simulink model "Lab_Loadcell"  (R2026a)
settings: Solver=FixedStepDiscrete  StartTime=0  StopTime=inf  FixedStep=0.001
undefined symbols (not defined in the file or in its folder): Blocking, Non
libraries: amg_usbconverter_n_connect_lib x2, dspstat3 x2, dspfdesign x1
settings Model: PauseTimes=10  Creator=pboon  LastModifiedBy=bocchichan

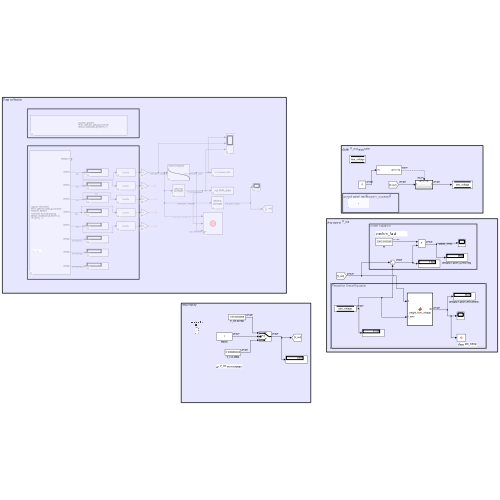
[thumbnail: Simulink's stored preview of the top-level diagram]
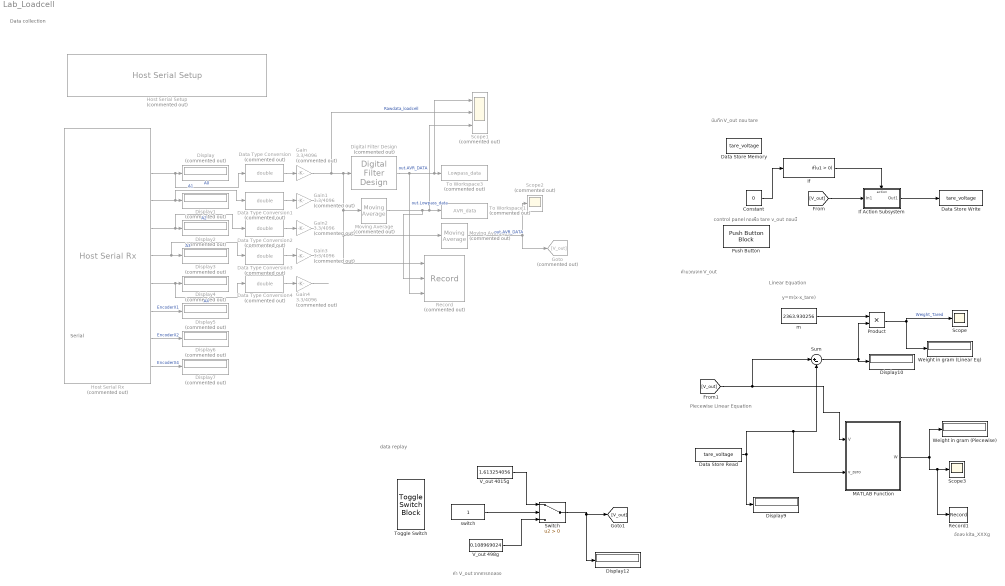
== system Lab_Loadcell ==
  note: อัดลง kita_XXXg
  note: ค่า V_out จากการทดลอง
  note: Data collection
  note: data replay
  note: Piecewise Linear Equation
  note: Linear Equation
  note: คำนวณจาก V_out
  note: control panel กดเพื่อ tare v_out ตอนนี้
  note: บันทึก V_out ตอน tare
  note: y=m(x-x_tare)
  note: Serial
  Constant : Constant  Value=0
  Data Store Memory : DataStoreMemory  DataStoreName=tare_voltage  WriteAfterWriteMsg=warning  ShowAdditionalParam=off  Dimensions=1
  Data Store Read : DataStoreRead  DataStoreName=tare_voltage  IndexOptions=Index vector (dialog)  Indices=1  OutputSizes=1
  Data Store Write : DataStoreWrite  DataStoreName=tare_voltage  IndexOptions=Index vector (dialog)  Indices=1  OutputSizes=1
  Data Type Conversion{,1..4} (5 alike) : DataTypeConversion  Commented=on  OutDataTypeStr=double  SaturateOnIntegerOverflow=off  RndMeth=Floor
  Digital Filter Design : dspfdesign/Digital Filter Design  Commented=on  mwdsp_browser_bugfix_var=off
  Display{,1..7} (8 alike) : Display  Commented=on
  Display10 : Display
  Display12 : Display
  Display9 : Display
  Gain{,1..4} (5 alike) : Gain  Commented=on  Gain=3.3/4096
  Goto : Goto  Commented=on  GotoTag=V_out
  Host Serial Rx : amg_usbconverter_n_connect_lib/Host Serial Rx  Commented=on  conf=rx  port=<auto>  baudrate=2000000  databits=8  parity=None  stopbit=1  flowcontrol=None  transfer=Non-Blocking  timeout=5  packetmode=Binary  enableinitialvalues=off  initialvalues=[]  binheader='25'  binterminator='4E 4E'  porttype_double=0  porttype_single=0  porttype_int8=0  porttype_uint8=0  porttype_int16=0  porttype_uint16=5  porttype_int32=0  porttype_uint32=3  asciiformat='%d,%f'  rx_asciiterminator="CRLF (0x0D 0x0A - \"\\r\\n\")"  tx_asciiterminator="CRLF (0x0D 0x0A - \"\\r\\n\")"  sampletime=0.001  enablecustomportlabel=off  cinputportlabel=0  coutputportlabel=A  portpinstr=0  blockid=HostSerialRx  inputporttype=[]  inputportwidth=[]  inputportlabel={}  outputporttype=[3 5 5 5 5 5 7 7 7]  outputportwidth=[1 1 1 1 1 1 1 1 1]  outputportlabel={'READY','uint16','uint16','uint16','uint16','uint16','uint32','uint32','uint32'}  compat=0  optionstring=[]  autoport='/dev/cu.debug-console'
  Host Serial Setup : amg_usbconverter_n_connect_lib/Host Serial Setup  Commented=on  conf=setup  port=<auto>  baudrate=2000000  databits=8  parity=None  stopbit=1  flowcontrol=None  transfer=Blocking  timeout=2  packetmode=Binary  initialvalues=[]  binheader='7E 7E'  binterminator='03 03'  porttype_double=0  porttype_single=1  porttype_int8=0  porttype_uint8=0  porttype_int16=0  porttype_uint16=0  porttype_int32=0  porttype_uint32=2  asciiformat='%d %u %x'  rx_asciiterminator="CRLF (0x0D 0x0A - \"\\r\\n\")"  tx_asciiterminator="CRLF (0x0D 0x0A - \"\\r\\n\")"  sampletime=-1  enablecustomportlabel=off  cinputportlabel=0  coutputportlabel=A  portpinstr=0  blockid=HostSerialSetup  inputporttype=[]  inputportwidth=[]  inputportlabel={}  outputporttype=[]  outputportwidth=[]  outputportlabel={}  compat=0  optionstring=[]  autoport='/dev/cu.debug-console'
  If : If  ShowElse=off
  If Action Subsystem : Subsystem  TreatAsAtomicUnit=on
  MATLAB Function : MATLAB Function  TreatAsAtomicUnit=on
  Moving Average : dspstat3/Moving Average  Commented=on  Method=Sliding window  ForgettingFactorPort=off  SpecifyWindowLength=on  WindowLengthSource=Property  MaxWindowLength=20  WindowLength=50  OverlapLength=49  AllowArbitraryInputLength=off  ForgettingFactor=0.9  SimulateUsing=Interpreted execution
  Moving Average1 : dspstat3/Moving Average  Commented=on  Method=Sliding window  ForgettingFactorPort=off  SpecifyWindowLength=on  WindowLengthSource=Property  MaxWindowLength=20  WindowLength=500  OverlapLength=499  AllowArbitraryInputLength=off  ForgettingFactor=0.9  SimulateUsing=Interpreted execution
  Product : Product
  Push Button : PushButtonBlock  ButtonText=Tare  IconOnColor=[0.0, 0.39215686274509803, 0.0]  IconOffColor=[0.0, 1.0, 0.0]  OffValue=0.000000
  Record : Record  Commented=on  NumPorts=3.0  FileSettingsInternal="{\"entries\":[{\"content\":{\"excelSettings\":{\"content\":{},\"type\":\"Streamout.ExcelSettings\"},\"parquetSettings\":{\"content\":{},\"type\":\"Streamout.ParquetSettings\"}},\"type\":\"Streamout.FileSettingStorage\",\"uuid\":\"\"}],\"packageUris\":[\"http:\\/\\/schema.mathworks.com\\/mf0\\/streamout_blocks\\/R2020a\"],\"version\":\"1.0\"}"  FrameSettings=[0, 0, 0]  Layout=[1 1]  SignalsInternal="{\"entries\":[{\"content\":{},\"type\":\"RecordBlkView.InputSignals\",\"uuid\":\"\"}],\"packageUris\":[\"http:\\/\\/schema.mathworks.com\\/mf0\\/streamout_blocks\\/R2020a\"],\"version\":\"1.0\"}"
  Record1 : Record  NumPorts=1.0  FileSettingsInternal="{\"entries\":[{\"content\":{\"excelSettings\":{\"content\":{},\"type\":\"Streamout.ExcelSettings\"},\"parquetSettings\":{\"content\":{},\"type\":\"Streamout.ParquetSettings\"}},\"type\":\"Streamout.FileSettingStorage\",\"uuid\":\"\"}],\"packageUris\":[\"http:\\/\\/schema.mathworks.com\\/mf0\\/streamout_blocks\\/R2020a\"],\"version\":\"1.0\"}"  FrameSettings=0  Layout=[1 1]  SignalsInternal="{\"entries\":[{\"content\":{\"signals\":[{\"content\":{\"blockPath\":[],\"dimensions\":[1],\"domain\":\"\",\"lineColor\":\"#64d413\",\"lineWidth\":2,\"port\":1,\"sid\":[\"\"],\"signalID\":1,\"signalName\":\"MATLAB Function\"},\"type\":\"RecordBlkView.Signal\",\"uuid\":\"\"}]},\"type\":\"RecordBlkView.InputSignals\",\"uuid\":\"\"}],\"packageUris\":[\"http:\\/\\/schema.mathworks.com\\/mf0\\/streamout_blocks\\/R2020a\"],\"version\":\"1.0\"}"
  Scope : Scope
  Scope1 : Scope  Commented=on  NumInputPorts=3
      settings: ActiveDisplayYMinimum=-0.43022761880155758  ActiveDisplayYMaximum=3.8720485692140194
  Scope2 : Scope  Commented=on
      settings: ActiveDisplayYMinimum=-1  ActiveDisplayYMaximum=1  DataLoggingVariableName=ScopeData2
  Scope3 : Scope
      settings: ActiveDisplayYMinimum=2695.10678668559  ActiveDisplayYMaximum=2920.0580839746385  DataLoggingVariableName=ScopeData3
  Sum : Sum  Inputs=|+-
  Switch : Switch  Criteria=u2 > Threshold  SaturateOnIntegerOverflow=off  InputSameDT=off
  To Workspace1 : ToWorkspace  Commented=on  VariableName=AVR_data  SaveFormat=Timeseries  SampleTime=-1
  To Workspace3 : ToWorkspace  Commented=on  VariableName=Lowpass_data  SaveFormat=Timeseries  SampleTime=-1
  Toggle Switch : ToggleSwitchBlock
  V_out 4015g : Constant  Value=1.613254056
  V_out 498g : Constant  Value=0.108969024
  Weight in gram (Linear Eq) : Display
  Weight in gram (Piecewise) : Display
  m : Constant  Value=2363.930256
  switch : Constant
  wires:
  Host Serial Rx/2 -> Data Type Conversion/1, Display/1  "A0"
  Host Serial Rx/3 -> Data Type Conversion1/1, Display1/1  "A1"
  Host Serial Rx/4 -> Data Type Conversion2/1, Display2/1  "A2"
  Host Serial Rx/5 -> Data Type Conversion3/1, Display3/1  "A3"
  Host Serial Rx/6 -> Data Type Conversion4/1, Display4/1  "A4"
  Host Serial Rx/7 -> Display5/1  "EncoderX1"
  Host Serial Rx/8 -> Display6/1  "EncoderX2"
  Host Serial Rx/9 -> Display7/1  "EncoderX4"
  Data Type Conversion/1 -> Gain/1
  Data Type Conversion1/1 -> Gain1/1
  Data Type Conversion2/1 -> Gain2/1
  Data Type Conversion4/1 -> Gain4/1
  Data Type Conversion3/1 -> Gain3/1
  Gain4/1 -> ?
  Gain3/1 -> ?
  Gain2/1 -> ?
  Gain1/1 -> ?
  Gain/1 -> Scope1/2, Record/1, Moving Average1/1, Moving Average/1, Digital Filter Design/1  "Rawdata_loadcell"
  Digital Filter Design/1 -> Record/3, Scope1/1, To Workspace3/1  "out.Lowpass_data"
  Moving Average/1 -> Record/2, Scope1/3, To Workspace1/1  "out.AVR_DATA"
  Constant/1 -> If/1
  If/1 -> If Action Subsystem/Action
  If Action Subsystem/1(Out1) -> Data Store Write/1
  [V_out] -> If Action Subsystem/1(In1)
  m/1 -> Product/1
  Sum/1 -> Display10/1, Product/2
  Product/1 -> Scope/1, Weight in gram (Linear Eq)/1  "Weight_Tared"
  switch/1 -> Switch/2
  Switch/1 -> Display12/1, [V_out]
  Moving Average1/1 -> Goto/1, Scope2/1  "out.AVR_DATA"
  MATLAB Function/1(W) -> Weight in gram (Piecewise)/1, Record1/1, Scope3/1
  Data Store Read/1 -> Display9/1, MATLAB Function/2(v_zero), Sum/2
  [V_out] -> MATLAB Function/1(V), Sum/1
  V_out 4015g/1 -> Switch/1
  V_out 498g/1 -> Switch/3

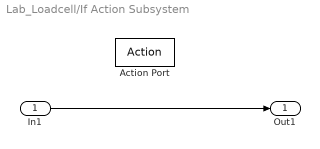
== system Lab_Loadcell/If Action Subsystem ==
  In1 : Inport
  Action Port : ActionPort  ActionPortLabel=if(u1 > 0)
  Out1 : Outport
  wires:
  In1/1 -> Out1/1

== matlab function Lab_Loadcell/MATLAB Function ==
  data: V input; W output; v_zero input
function W = weight_from_voltage(V, v_zero)
%WEIGHT_FROM_VOLTAGE  Calibration curve: grams from load-cell filter voltage.
%   W = weight_from_voltage(V)            gross weight at voltage V (volts)
%   W = weight_from_voltage(V, v_zero)    net weight, tared at voltage v_zero
%   V may be a scalar or an array of any size; the output matches its size.

%   Tare subtracts in GRAM space:  W = f(V) - f(v_zero).
%   Do NOT use f(V - v_zero): the breakpoints are absolute volts and the curve
%   does not pass through the origin, so subtracting volts slides the reading
%   along the curve instead of moving its zero. With v_zero = 0.108853 V
%   (the 498 g point) and V = 2.045659 V (5014 g), gram space gives the correct
%   4516 g net; volt space gives 4761 g, i.e. +245 g.

    V_bp = [0.02034129238; 0.10885345236; 0.32732078439; 0.53873194403; ...
            0.74910236319; 0.96156417441; 1.18144135240; 1.39864106487; ...
            1.61317916379; 1.83031967722; 2.04565942028; 2.25816807979; ...
            2.47800513007; 2.68192913214; 2.89197483609; 3.07765532174];   % volts
    W_tb = [0; 498; 1026; 1525; 2021; 2521; 3024; 3521; ...
            4015; 4513; 5014; 5512; 6013; 6511; 7000; 7500];               % grams

    if nargin < 2
        v_zero = V_bp(1);                 % no tare: the 0 g point reads 0 g
    end

    W = curve(V_bp, W_tb, V) - curve(V_bp, W_tb, v_zero);
end

function w = curve(V_bp, W_tb, v)
    w = interp1(V_bp, W_tb, min(max(v, V_bp(1)), V_bp(end)));
end
